simulink model "RadioReceiver"  (R2017b)
settings: Solver=FixedStepDiscrete  StartTime=0.0  StopTime=10.0  RelTol=1e-3
InitFcn:
  | barker = comm.BarkerCode('SamplesPerFrame', 28, 'Length', 11);
  | seq = barker()+1;
  | M = 4;
  | hPSKModTrain   = comm.PSKModulator(M, ...
  |     'PhaseOffset',pi/4, ...
  |     'SymbolMapping','Binary');
  | xPreambleSeq = hPSKModTrain(seq);
  | 
  | 
  | %%%%%%%%%%%%
  | 
  | % AGC Preamble
  | reps = 5;
  | barker = comm.BarkerCode('SamplesPerFrame', 16, 'Length', 13);
  | seq = barker()+1;
  | %preamble = zeros(16*reps,1);
  | preambleFull = repmat(seq,reps,1);
  | rctFilt = comm.RaisedCosineTransmitFilter('FilterSpanInSymbols', 128,...
  | 'RolloffFactor',0.5,...
  | 'OutputSamplesPerSymbol',4);
  | preambleFullFilt = rctFilt(preambleFull);
  | 
  | %%%%%%%%%%%%
  | 
  | RadioSampleRate = 1e6;
  | %RadioSampleRate = 20e6;
  | RadioFrameLength = 1e5;
  | 
  | VibertiTracebackLength = 34+0;
  | numTrainingSamples = 250;
  | crc32Poly = [1 0 0 0 0 0 1 0 0 1 1 0 0 0 0 0 1 0 0 0 1 1 1 0 1 1 0 1 1 0 1 1 1];
  | crcDecodeLag = length(crc32Poly)-1+2;
  | 
  | %%%%%%%%%%%%
  | 
  | beta = 0.5;
  | span = 8;
  | sps = 4;
  | filterGain = 1;
  | coeff = rcosdesign(beta, span, sps, 'sqrt')*filterGain;
  | 
  | %%%%%%%%%%%%
  | 
  | samplesPerSymbol = 4;
  | maxPacketBits = 8*1500;
  | bItsPerSymbol = 2;
  | CodeRate = 2;
  | tailSymbols = 40;
  | maxPayloadSymbols = maxPacketBits*CodeRate/bItsPerSymbol+tailSymbols;
libraries: commsource2 x1, RxFloatingPointLibrary x1
settings Model: DataTypeOverride=Off  MinMaxOverflowLogging=MinMaxAndOverflow  FPTRunName=NoOverride  Creator=tcollins  LastModifiedBy=tcollins
settings DataIOCC: SaveOutput=off  SaveTime=off
settings OptimizationCC: BlockReduction=off  ConditionallyExecuteInputs=off  DefaultParameterBehavior=Inlined
settings DebuggingCC: AlgebraicLoopMsg=error  SingleTaskRateTransMsg=error
settings HardwareCC: ProdBitPerPointer=32  ProdBitPerSizeT=32  ProdBitPerPtrDiffT=32  ProdLargestAtomicFloat=None  ProdIntDivRoundTo=Undefined  ProdEndianess=Unspecified  ProdWordSize=32  ProdHWDeviceType=ASIC/FPGA->ASIC/FPGA  ProdEqTarget=off
settings CodeAppCC: StateflowObjectComments=on
settings SimscapeCC: SimscapeNormalizeSystem=off

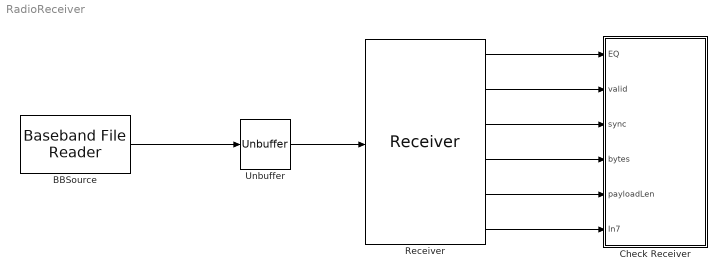
== system RadioReceiver ==
  BBSource : commsource2/Baseband File Reader  Filename=IQ_baseline.bb  InheritSampleTimeFromFile=off  SampleTime=100000/(RadioSampleRate)  SamplesPerFrame=100000  CyclicRepetition=on  FileEndOutputPort=off  SimulateUsing=Interpreted execution
      settings: SourceProductName=Communications System Toolbox  SourceProductBaseCode=CM
  Check Receiver : Subsystem
  Receiver : RxFloatingPointLibrary/Receiver
  Unbuffer : Unbuffer
  wires:
  BBSource/1 -> Unbuffer/1
  Unbuffer/1 -> Receiver/1
  Receiver/1 -> Check Receiver/1(EQ)
  Receiver/6 -> Check Receiver/6(In7)
  Receiver/2 -> Check Receiver/2(valid)
  Receiver/3 -> Check Receiver/3(sync)
  Receiver/4 -> Check Receiver/4(bytes)
  Receiver/5 -> Check Receiver/5(payloadLen)

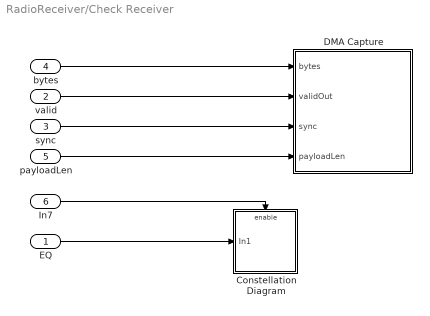
== system RadioReceiver/Check Receiver ==
  EQ : Inport
  valid : Inport  Port=2
  sync : Inport  Port=3
  bytes : Inport  Port=4
  payloadLen : Inport  Port=5
  In7 : Inport  Port=6
  Constellation Diagram : Subsystem
  DMA Capture : MATLAB Function  TreatAsAtomicUnit=on
  wires:
  EQ/1 -> Constellation Diagram/1(In1)
  In7/1 -> Constellation Diagram/Enable
  bytes/1 -> DMA Capture/1(bytes)
  valid/1 -> DMA Capture/2(validOut)
  sync/1 -> DMA Capture/3(sync)
  payloadLen/1 -> DMA Capture/4(payloadLen)

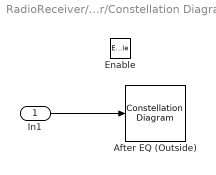
== system RadioReceiver/Check Receiver/Constellation Diagram ==
  In1 : Inport
  Enable : EnablePort
  After EQ (Outside) : ConstellationDiagram
  wires:
  In1/1 -> After EQ (Outside)/1

== matlab function RadioReceiver/Check Receiver/DMA Capture ==
  data: bytes input; validOut input; sync input; payloadLen input
function fcn(bytes, validOut, sync, payloadLen)

persistent frameBuffer byteCounter fullPayloadBits

if isempty(frameBuffer)
    frameBuffer = false(2^16,1);
    byteCounter = 0;
    fullPayloadBits = uint16(0);
end

if validOut
    if sync
        byteCounter = 32;
        frameBuffer(1:byteCounter) = bitget(bytes,1:32);
        fullPayloadBits = uint16(payloadLen*8);
        
    elseif byteCounter<fullPayloadBits
        frameBuffer(byteCounter+1:byteCounter+32) = bitget(bytes,1:32);
        byteCounter = byteCounter + 32;
    else
        if bytes>0
            %disp('CRC Error (Outside)');
        else
            %disp('Frame passed CRC (Outside)');
        end
    end
end
